simulink model "aeroblk_wf_3dof"  (Simulink 6.0)
settings: Solver=ode45  StartTime=0.0  StopTime=10  FixedStep=0.01  MaxStep=0.02  RelTol=1e-3
PreLoadFcn:
  | aeroblk_wf_3dof_data;
undefined symbols (not defined in the file or in its folder): rad, s
libraries: vrlib x6, aeroblk_lib_wf_3dof x3, aerolibconvert x2, simulink x1
CloseFcn:
  | clear wf_B3 wf_H wf_Q2 wf_Q4 wf_alpha wf_alpha2 wf_alphaa wf_c wf_cd wf_cg wf_cl wf_cls wf_cm wf_cp_e wf_gravity wf_incidence wf_weight wf_z1 wf_z2 wf_z3 wf_inertia wf_sref wf_w2e wf_q;
  | 
  | clear ports tempFixPtSimRanges
settings Model: Creator=The MathWorks Inc.  LastModifiedBy=batserve  ExtModeAutoUpdateStatusClock=off
settings DataIOCC: SaveOutput=off  SaveTime=off  SignalLoggingName=sigsOut
settings DebuggingCC: CheckExecutionContextPreStartOutputMsg=on  CheckExecutionContextRuntimeOutputMsg=on  SolverPrmCheckMsg=none
settings HardwareCC: TargetUnknown=on

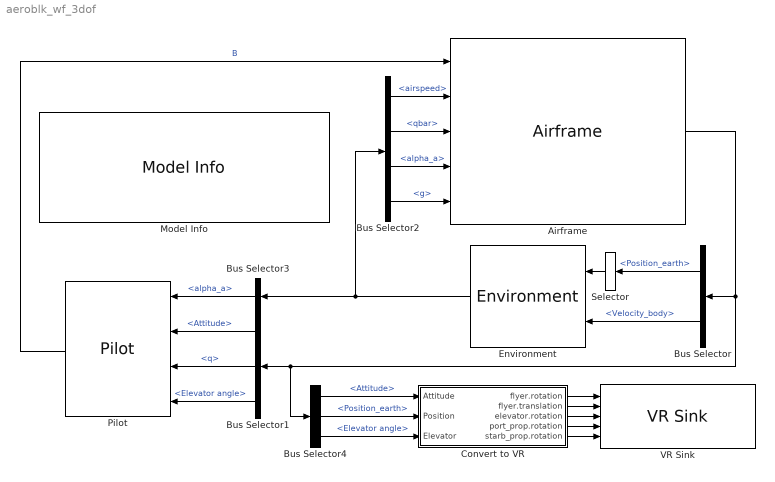
== system aeroblk_wf_3dof ==
  Airframe : aeroblk_lib_wf_3dof/Airframe
  Bus Selector : BusSelector  Orientation=left  DialogController=Simulink.DDGSource_Bus  OutputSignals=Position_earth,Velocity_body
  Bus Selector1 : BusSelector  Orientation=left  DialogController=Simulink.DDGSource_Bus  OutputSignals=Attitude,q,Elevator angle
  Bus Selector2 : BusSelector  DialogController=Simulink.DDGSource_Bus  OutputSignals=airspeed,qbar,alpha_a,g
  Bus Selector3 : BusSelector  Orientation=left  DialogController=Simulink.DDGSource_Bus  OutputSignals=alpha_a
  Bus Selector4 : BusSelector  DialogController=Simulink.DDGSource_Bus  OutputSignals=Attitude,Position_earth,Elevator angle
  Convert to VR : Subsystem  PropExecContextAcrossSSBoundary=on
      mask Display:
      | port_label('input',1,'Altitude')
      | port_label('input',2,'Position')
      | port_label('input',3,'Elevator')
      | port_label('output',1,'flyer.rotation')
      | port_label('output',2,'flyer.translation')
      | port_label('output',3,'elevator.rotation')
      | port_label('output',4,'port_prop.rotation')
      | port_label('output',5,'starb_prop.rotation')
  Environment : aeroblk_lib_wf_3dof/Environment  Orientation=left
  Model Info : simulink/Model-Wide Utilities/Model Info  InitialBlockCM=None  BlockCM=None  Frame=on  DisplayStringWithTags=|  HorizontalTextAlignment=Center  LeftAlignmentValue=0.5  SourceBlockDiagram=aeroblk_wf_3dof  TagMaxNumber=20
      | 1903 Wright Flyer
      | based on 
      | Hooven, Frederick J., "Longitudinal 
      | Dynamics of the Wright Brothers' Early Flyers 
      | 'A Study in Computer Simulation of Flight'", 
      | from The Wright Flyer An Engineering Perspective 
      | edited by Howard S. Wolko, 1987.%<Description>
  Pilot : aeroblk_lib_wf_3dof/Pilot  Orientation=left
  Selector : Selector  Orientation=left  Elements=2  InputPortWidth=2
  VR Sink : vrlib/VR Sink  SampleTime=-1  ViewEnable=on  RemoteChange=off  RemoteView=off  FieldsWritten=flyer.rotation.4.1.double#flyer.translation.3.1.double#canard.rotation.4.1.double#portpropeller.rotation.4.1.double#starboardpropeller.rotation.4.1.double  WorldFileName=aeroblk_wf_3dof.wrl  AutoView=on  FigureProperties="{'Position', 'Name', 'Viewpoint', 'CameraBound', 'CameraDirection', 'CameraPosition', 'CameraUpVector', 'ZoomFactor', 'Antialiasing', 'Headlight', 'Lighting', 'NavPanel', 'StatusBar', 'ToolBar', 'Textures', 'Transparency', 'Wireframe', 'NavZones', 'NavMode', 'NavSpeed', 'Record2DCompressMethod', 'Record2DCompressQuality', 'Record2D', 'Record2DFileName'; [0.0000000000000000e+00   6.0000000000000000e+01   5.8000000000000000e+02   2.8800000000000000e+02], '1903 Wright Flyer', 'Side-Rear View', 'on', [0.0000000000000000e+00   0.0000000000000000e+00  -1.0000000000000000e+00], [0.0000000000000000e+00   0.0000000000000000e+00   0.0000000000000000e+00], [0.0000000000000000e+00   1.0000000000000000e+00   0.0000000000000000e+00], [1.0000000000000000e+00], 'off', 'on', 'on', 'halfbar', 'on', 'on', 'on', 'on', 'off', 'off', 'walk', 'normal', 'auto', [7.5000000000000000e+01], 'off', '%f_anim_%n.avi'}"
  wires:
  Environment/1 -> Bus Selector2/1, Bus Selector3/1
  Pilot/1 -> Airframe/1  "B"
  Airframe/1 -> Bus Selector/1, Bus Selector1/1, Bus Selector4/1
  Bus Selector/1 -> Selector/1  "<Position_earth>"
  Bus Selector/2 -> Environment/2  "<Velocity_body>"
  Selector/1 -> Environment/1
  Bus Selector1/1 -> Pilot/2  "<Attitude>"
  Bus Selector1/2 -> Pilot/3  "<q>"
  Bus Selector1/3 -> Pilot/4  "<Elevator angle>"
  Bus Selector2/1 -> Airframe/2  "<airspeed>"
  Bus Selector2/2 -> Airframe/3  "<qbar>"
  Bus Selector2/3 -> Airframe/4  "<alpha_a>"
  Bus Selector2/4 -> Airframe/5  "<g>"
  Bus Selector3/1 -> Pilot/1  "<alpha_a>"
  Bus Selector4/2 -> Convert to VR/2(Position)  "<Position_earth>"
  Bus Selector4/1 -> Convert to VR/1(Attitude)  "<Attitude>"
  Bus Selector4/3 -> Convert to VR/3(Elevator)  "<Elevator angle>"
  Convert to VR/1(flyer.rotation) -> VR Sink/1
  Convert to VR/2(flyer.translation) -> VR Sink/2
  Convert to VR/3(elevator.rotation) -> VR Sink/3
  Convert to VR/4(port_prop.rotation) -> VR Sink/4
  Convert to VR/5(starb_prop.rotation) -> VR Sink/5

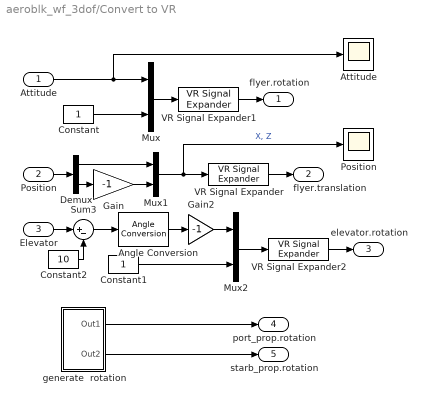
== system aeroblk_wf_3dof/Convert to VR ==
  Attitude : Inport  Port=1  LatchInput=off
  Position : Inport  Port=2  LatchInput=off
  Elevator : Inport  Port=3  LatchInput=off
  Angle Conversion : aerolibconvert/Angle Conversion  IU=deg  OU=rad
  "Attitude " : Scope
      settings: TimeRange=3  YMin=-0.25  YMax=-0.05
  Constant : Constant
  Constant1 : Constant
  Constant2 : Constant  Value=10
  Demux : Demux  Outputs=2
  Gain : Gain  Gain=-1  SaturateOnIntegerOverflow=on
  Gain2 : Gain  Gain=-1  SaturateOnIntegerOverflow=on
  Mux : Mux  Inputs=2
  Mux1 : Mux  Inputs=2
  Mux2 : Mux  Inputs=2
  "Position " : Scope
      settings: TimeRange=3  YMin=-3.05311e-16  YMax=100
  Sum3 : Sum  Inputs=|+-  SaturateOnIntegerOverflow=on
  VR Signal Expander : vrlib/VR Signal Expander  outwidth=3  outidx=[3 2]
  VR Signal Expander1 : vrlib/VR Signal Expander  outwidth=4  outidx=[4 1]
  VR Signal Expander2 : vrlib/VR Signal Expander  outwidth=4  outidx=[4 1]
  generate  rotation : Subsystem  PropExecContextAcrossSSBoundary=on
  flyer.rotation : Outport
  flyer.translation : Outport  Port=2
  elevator.rotation : Outport  Port=3
  port_prop.rotation : Outport  Port=4
  starb_prop.rotation : Outport  Port=5
  wires:
  Mux/1 -> VR Signal Expander1/1
  Constant/1 -> Mux/2
  Attitude/1 -> Mux/1, "Attitude "/1
  VR Signal Expander1/1 -> flyer.rotation/1
  Position/1 -> Demux/1
  VR Signal Expander/1 -> flyer.translation/1
  generate  rotation/1(Out1) -> port_prop.rotation/1
  generate  rotation/2(Out2) -> starb_prop.rotation/1
  Elevator/1 -> Sum3/1
  Angle Conversion/1 -> Gain2/1
  Mux1/1 -> VR Signal Expander/1, "Position "/1  "X, Z"
  Demux/2 -> Gain/1
  Gain/1 -> Mux1/2
  Demux/1 -> Mux1/1
  VR Signal Expander2/1 -> elevator.rotation/1
  Mux2/1 -> VR Signal Expander2/1
  Constant1/1 -> Mux2/2
  Gain2/1 -> Mux2/1
  Sum3/1 -> Angle Conversion/1
  Constant2/1 -> Sum3/2

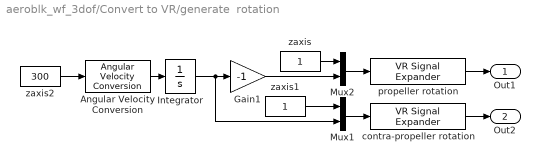
== system aeroblk_wf_3dof/Convert to VR/generate  rotation ==
  Angular Velocity Conversion : aerolibconvert/Angular Velocity Conversion  IU=rpm  OU=rad/s
  Gain1 : Gain  Gain=-1  SaturateOnIntegerOverflow=on
  Integrator : Integrator
  Mux1 : Mux  Inputs=2
  Mux2 : Mux  Inputs=2
  contra-propeller rotation : vrlib/VR Signal Expander  outwidth=4  outidx=[3 4]
  propeller rotation : vrlib/VR Signal Expander  outwidth=4  outidx=[3 4]
  zaxis : Constant
  zaxis1 : Constant
  zaxis2 : Constant  Value=300
  Out1 : Outport
  Out2 : Outport  Port=2
  wires:
  zaxis2/1 -> Angular Velocity Conversion/1
  contra-propeller rotation/1 -> Out2/1
  propeller rotation/1 -> Out1/1
  Gain1/1 -> Mux2/2
  zaxis1/1 -> Mux1/1
  Mux1/1 -> contra-propeller rotation/1
  Mux2/1 -> propeller rotation/1
  zaxis/1 -> Mux2/1
  Integrator/1 -> Mux1/2, Gain1/1
  Angular Velocity Conversion/1 -> Integrator/1
